simulink model "test_rfdcmask_zcu216"  (R2020b)
settings: Solver=VariableStepAuto  StartTime=0.0  StopTime=10.0  RelTol=1e-3
undefined symbols (not defined in the file): es1
libraries: xbsIndex_r4 x201, casper_library_misc x2
(part 1 of 4)
settings Model: Creator=mcb  LastModifiedBy=mcb
settings DataIOCC: ReturnWorkspaceOutputs=off
settings DebuggingCC: ArithmeticOperatorsInVariantConditions=warning
settings SFSimCC: CustomCodeUndefinedFunction=UseInterfaceOnly

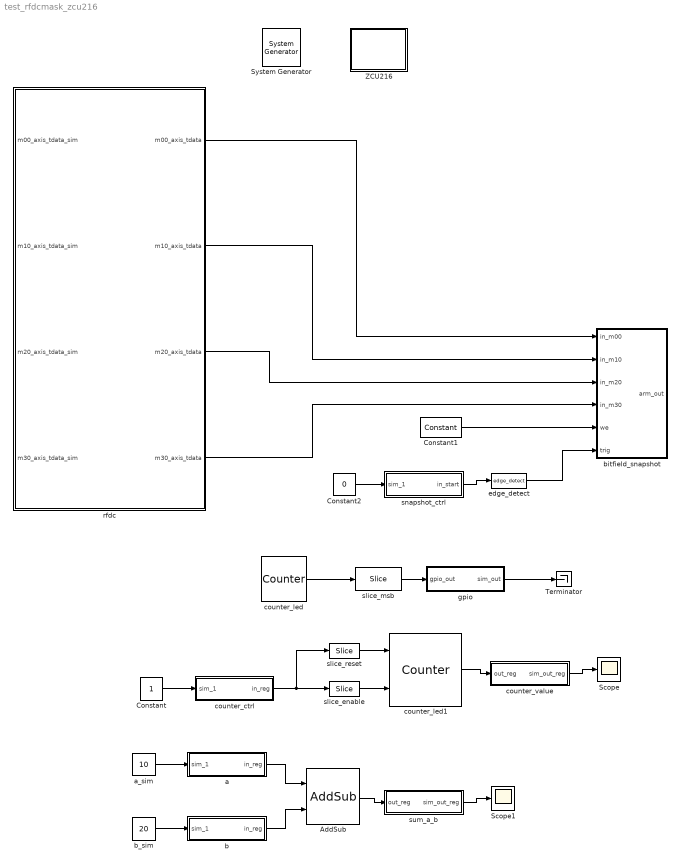
== system test_rfdcmask_zcu216 ==
  " System Generator" : xbsIndex_r4/ System Generator  Tag=genX  xilinxfamily=zynquplusRFSOCes1  part=xczu49dr  speed=-2-e-es1  package=ffvf1760  synthesis_tool=XST  clock_wrapper=Clock Enables  directory=/home/mcb/git/casper/mlib_devel/jasper_library/test_models/test_rfdcmask_zcu216/sysgen  proj_type=Vivado  Synth_file=Vivado Synthesis Defaults  Impl_file=Vivado Implementation Defaults  testbench=off  simulink_period=1  sysclk_period=4  dcm_input_clock_period=10  incr_netlist=off  trim_vbits=Everywhere in SubSystem  dbl_ovrd=According to Block Masks  core_generation=According to Block Masks  run_coregen=off  deprecated_control=off  eval_field=0  block_type=sysgen
  AddSub : xbsIndex_r4/AddSub  mode=Addition  use_carryin=off  use_carryout=off  en=off  latency=0  precision=User Defined  arith_type=Unsigned  n_bits=32  bin_pt=0  quantization=Truncate  overflow=Saturate  use_behavioral_HDL=off  hw_selection=Fabric  pipelined=off  dbl_ovrd=off  block_type=addsub
  Constant : Constant
  Constant1 : xbsIndex_r4/Constant  const=1.0  gui_display_data_type=Boolean  arith_type=Boolean  n_bits=16  bin_pt=14  preci_type=Single  exp_width=8  frac_width=24  explicit_period=on  period=1  equ=P=C  opselect=C  inp2=PCIN>>17  opr=+  inp1=P  carry=CIN  dbl_ovrd=off  block_type=constant
  Constant2 : Constant  Value=0
  Scope : Scope
  Scope1 : Scope
  Terminator : Terminator
  ZCU216 : Subsystem  Tag=xps:xsg  mask(xsg core config){hw_sys=ZCU216:xczu49dr, clk_src=adc_clk, clk_rate=250, pl_clk_rate=125, sample_period=1, synthesis_tool=XST}
      mask prompts: hw_sys "Hardware Platform"; clk_src "User IP Clock source"; clk_rate "User IP Clock Rate (MHz)"; pl_clk_rate "RFPLL PL Clock Rate (MHz)"; sample_period "Sample Period"; synthesis_tool "Synthesis Tool:"
      mask help:
      | The XSG Core Config block is used to configure the System Generator design
      | for the casper_xps toolflow. Settings here are used to configure the
      | Xilinx System Generator block parameters automatically, and control toolflow
      | script  execution. It needs to be at the top level of all designs being compiled
      | with the casper_xps toolflow.
      mask init:
      | xps_xsg_zcu216_conf_mask;
      mask Help: eval('xlWeb([getenv(''MLIB_ROOT''), ''\doc\html\sys_xsg_core_config\sys_xsg_core_config.html''])')
      mask TypeOptions hw_sys: ZCU216:xczu49dr
      mask TypeOptions clk_src: adc_clk
      mask TypeOptions synthesis_tool: Leonardo Spectrum | Synplify | Synplify Pro | XST
      mask Display: fprintf(['ZCU216']);
  a : Subsystem  Tag=xps:sw_reg  AncestorBlock=xps_library/Memory/software_register  mask(swreg){io_dir=From Processor, io_delay=0, init_val=0, sample_period=1, names=reg, bitwidths=32, bin_pts=0, arith_types=0, sim_port=on, show_format=off}
      mask prompts: io_dir "I/O direction"; io_delay "I/O delay"; init_val "Initial Value"; sample_period "Sample period"; names "Bitfield names [msb...lsb]"; bitwidths "Bitfield widths"; bin_pts "Bitfield binary pts"; arith_types "Bitfield types, ufix=0, fix=1, bool=2"; sim_port "Provide sim input/output?"; show_format "Print format string?"
      mask help: A 32-bit software-accessible register. Can be divided into bitfields of varying widths and types using the fields in the block mask.
      mask init:
      | swreg_init(gcb)
      settings: AttributesFormatString=1input
      mask TypeOptions io_dir: To Processor | From Processor
      mask Callback io_dir:
      | mask_enables = get_param(gcb, 'MaskEnables');
      | mask_names = get_param(gcb, 'MaskNames');
      | if strcmp(get_param(gcb, 'io_dir'), 'To Processor'),
      |     mask_enables{ismember(mask_names, 'sample_period')} = 'off';
      | else
      |     mask_enables{ismember(mask_names, 'sample_period')} = 'on';
      | end
      | set_param(gcb, 'MaskEnables', mask_enables);
      mask DialogControl ParameterTabVar0 Prompt: Setup
  a_sim : Constant  Value=10
  b : Subsystem  Tag=xps:sw_reg  AncestorBlock=xps_library/Memory/software_register  mask(swreg){io_dir=From Processor, io_delay=0, init_val=0, sample_period=1, names=reg, bitwidths=32, bin_pts=0, arith_types=0, sim_port=on, show_format=off}
      mask prompts: io_dir "I/O direction"; io_delay "I/O delay"; init_val "Initial Value"; sample_period "Sample period"; names "Bitfield names [msb...lsb]"; bitwidths "Bitfield widths"; bin_pts "Bitfield binary pts"; arith_types "Bitfield types, ufix=0, fix=1, bool=2"; sim_port "Provide sim input/output?"; show_format "Print format string?"
      mask help: A 32-bit software-accessible register. Can be divided into bitfields of varying widths and types using the fields in the block mask.
      mask init:
      | swreg_init(gcb)
      settings: AttributesFormatString=1input
      mask TypeOptions io_dir: To Processor | From Processor
      mask Callback io_dir:
      | mask_enables = get_param(gcb, 'MaskEnables');
      | mask_names = get_param(gcb, 'MaskNames');
      | if strcmp(get_param(gcb, 'io_dir'), 'To Processor'),
      |     mask_enables{ismember(mask_names, 'sample_period')} = 'off';
      | else
      |     mask_enables{ismember(mask_names, 'sample_period')} = 'on';
      | end
      | set_param(gcb, 'MaskEnables', mask_enables);
      mask DialogControl ParameterTabVar0 Prompt: Setup
  b_sim : Constant  Value=20
  bitfield_snapshot : Subsystem  Tag=casper:bitsnap  AncestorBlock=casper_library_scopes/bitfield_snapshot  mask(bitsnap){io_names=[m00 m10 m20 m30], io_widths=[16 16 16 16], io_bps=[0 0 0 0], io_types=[1 1 1 1], show_format=on, snap_storage=bram, snap_dram_dimm=2, snap_dram_clock=250, snap_nsamples=12, snap_data_width=64, snap_offset=off, snap_circap=off, snap_value=off, snap_ext_arm=off, snap_ext_circ=off, snap_provide_outputs=on, snap_use_dsp48=on, snap_delay=2, extra_names=[c d], extra_widths=[30 2], extra_bps=[0 0], extra_types=[0 0]}
      mask prompts: io_names "Names [msb...lsb]"; io_widths "Bitwidths [msb...lsb]"; io_bps "Binary pts [msb...lsb]"; io_types "Data types [msb...lsb], ufix=0, fix=1, bool=2"; show_format "Print format string?"; snap_storage "Storage medium"; snap_dram_dimm "DRAM dimm"; snap_dram_clock "DRAM clock rate"; snap_nsamples "Number of Samples (2^?)"; snap_data_width "Data width"; snap_offset "Start delay support"; snap_circap "Circular capture support"; snap_value "Extra value capture support"; snap_ext_arm "External arm support"; snap_ext_circ "External circular capture support"; snap_provide_outputs "Provide outputs"; snap_use_dsp48 "Use DSP48s to implement counters"; snap_delay "Pre-snapshot delay"; extra_names "Names [msb...lsb]"; extra_widths "Widths [msb...lsb]"; extra_bps "Binary pts [msb...lsb]"; extra_types "Data types [msb...lsb], ufix=0, fix=1, bool=2"
      mask help:
      | A wrapped snapshot block. Allows specification of inputs to a snapblock word so the toolflow can automatically set up the scope.
      | See documentation for snapshot for explanation of parameters.
      mask init:
      | bitsnap_init(gcb);
      settings: AttributesFormatString=|
      | snap(4):f16.0,f16.0,f16.0,f16.0 = 64 bits\n64 wide, 4096 deep
      | debugID: 125644504
      mask TypeOptions snap_storage: bram | dram
      mask Callback snap_storage: bitsnap_callback();
      mask TypeOptions snap_dram_dimm: 1 | 2 | 3 | 4
      mask TypeOptions snap_dram_clock: 200 | 250 | 266 | 300 | 333
      mask TypeOptions snap_data_width: 8 | 16 | 32 | 64 | 128
      mask Callback snap_value: bitsnap_callback();
      mask Callback snap_ext_arm: bitsnap_callback();
      mask Callback snap_ext_circ: bitsnap_callback();
      mask Callback snap_provide_outputs: bitsnap_callback();
      mask DialogControl ParameterTabVar0 Prompt: Inputs
      mask DialogControl ParameterTabVar01 Prompt: Snapshot
      mask DialogControl ParameterTabVar012 Prompt: Extra Value
  counter_ctrl : Subsystem  Tag=xps:sw_reg  AncestorBlock=xps_library/Memory/software_register  mask(swreg){io_dir=From Processor, io_delay=0, init_val=0, sample_period=1, names=reg, bitwidths=32, bin_pts=0, arith_types=0, sim_port=on, show_format=off}
      mask prompts: io_dir "I/O direction"; io_delay "I/O delay"; init_val "Initial Value"; sample_period "Sample period"; names "Bitfield names [msb...lsb]"; bitwidths "Bitfield widths"; bin_pts "Bitfield binary pts"; arith_types "Bitfield types, ufix=0, fix=1, bool=2"; sim_port "Provide sim input/output?"; show_format "Print format string?"
      mask help: A 32-bit software-accessible register. Can be divided into bitfields of varying widths and types using the fields in the block mask.
      mask init:
      | swreg_init(gcb)
      settings: AttributesFormatString=1input
      mask TypeOptions io_dir: To Processor | From Processor
      mask Callback io_dir:
      | mask_enables = get_param(gcb, 'MaskEnables');
      | mask_names = get_param(gcb, 'MaskNames');
      | if strcmp(get_param(gcb, 'io_dir'), 'To Processor'),
      |     mask_enables{ismember(mask_names, 'sample_period')} = 'off';
      | else
      |     mask_enables{ismember(mask_names, 'sample_period')} = 'on';
      | end
      | set_param(gcb, 'MaskEnables', mask_enables);
      mask DialogControl ParameterTabVar0 Prompt: Setup
  counter_led : xbsIndex_r4/Counter  cnt_type=Free Running  cnt_to=Inf  operation=Up  start_count=0  cnt_by_val=1  arith_type=Unsigned  n_bits=28  bin_pt=0  load_pin=off  rst=off  en=off  explicit_period=on  period=1  use_behavioral_HDL=off  implementation=Fabric  dbl_ovrd=off  block_type=counter
  counter_led1 : xbsIndex_r4/Counter  cnt_type=Free Running  cnt_to=Inf  operation=Up  start_count=0  cnt_by_val=1  arith_type=Unsigned  n_bits=32  bin_pt=0  load_pin=off  rst=on  en=on  explicit_period=on  period=1  use_behavioral_HDL=off  implementation=Fabric  dbl_ovrd=off  block_type=counter
  counter_value : Subsystem  Tag=xps:sw_reg  AncestorBlock=xps_library/Memory/software_register  mask(swreg){io_dir=To Processor, io_delay=0, init_val=0, sample_period=1, names=reg, bitwidths=32, bin_pts=0, arith_types=0, sim_port=on, show_format=off}
      mask prompts: io_dir "I/O direction"; io_delay "I/O delay"; init_val "Initial Value"; sample_period "Sample period"; names "Bitfield names [msb...lsb]"; bitwidths "Bitfield widths"; bin_pts "Bitfield binary pts"; arith_types "Bitfield types, ufix=0, fix=1, bool=2"; sim_port "Provide sim input/output?"; show_format "Print format string?"
      mask help: A 32-bit software-accessible register. Can be divided into bitfields of varying widths and types using the fields in the block mask.
      mask init:
      | swreg_init(gcb)
      settings: AttributesFormatString=1output
      mask TypeOptions io_dir: To Processor | From Processor
      mask Callback io_dir:
      | mask_enables = get_param(gcb, 'MaskEnables');
      | mask_names = get_param(gcb, 'MaskNames');
      | if strcmp(get_param(gcb, 'io_dir'), 'To Processor'),
      |     mask_enables{ismember(mask_names, 'sample_period')} = 'off';
      | else
      |     mask_enables{ismember(mask_names, 'sample_period')} = 'on';
      | end
      | set_param(gcb, 'MaskEnables', mask_enables);
      mask DialogControl ParameterTabVar0 Prompt: Setup
  edge_detect : casper_library_misc/edge_detect  edge=Rising  polarity=Active High  x_in=[0 0.08 0.08 0.16 0.16 0.24 0.24 0.32 0.32 0.4]  y_in="[-1 -1  1  1  1  1  1  1  1  1]"  x_out=[0.6 0.68 0.68 0.76 0.76 0.84 0.84 0.92 0.92 1]  y_out="[-1 -1  1  1 -1 -1 -1 -1 -1 -1]"
  gpio : Subsystem  Tag=xps:gpio  AncestorBlock=xps_library/IO/gpio  mask(gpio){io_group_params_forwarded=on, io_group=ROACH2:led, io_group_real=led, io_group_custom=0, io_dir=out, arith_type=Boolean, bitwidth=1, bin_pt=0, bit_index=0, sample_period=1, use_single_ended=off, use_ddr=off, reg_iob=on, reg_clk_phase=0, termination=None}
      mask prompts: io_group_params_forwarded "Have the io_group params been forwarded yet?"; io_group "I/O group"; io_group_real "I/O group"; io_group_custom "Custom I/O group"; io_dir "I/O direction"; arith_type "Data Type"; bitwidth "Data bitwidth"; bin_pt "Data binary point"; bit_index "GPIO bit index"; sample_period "Sample period"; use_single_ended "Use as single-ended"; use_ddr "Use DDR"; reg_iob "Pack register in the pad"; reg_clk_phase "Register clock phase"; termination "Termination method"
      mask help:
      | GPIO interfaces for CASPER hardware.
      |
      | For usage of LEDs on SKARAB boards, please note that the board will boot into 'BSP mode' by default. To change the control of the Front Panel LEDs to your design, execute the command 'control_front_panel_leds_write()' on your SKARAB CASPERFPGA object via the transport layer.
      |
      | For more information please click help below.
      mask init:
      | gpio_mask;
      mask Help: If you've come here for more help, unfortunately I'm going to direct you to the ska-sa/casperfpga wiki. The documentation at https://github.com/ska-sa/casperfpga/wiki/SKARAB-Front-Panel-LED-Manager outlines the signals that are used to control the SKARAB's Front Panel LEDs by default, and the mechanism by which you can switch control to the DSP Design.
      mask TypeOptions io_group: ROACH:aux0_clk | ROACH:aux1_clk | ROACH:led | ROACH:gpioa | ROACH:gpioa_oe_n | ROACH:gpiob | ROACH:gpiob_oe_n | ROACH:qsh | ROACH:zdok0 | ROACH:zdok1 | ROACH2:aux_clk | ROACH2:led | ROACH2:gpio | ROACH2:qsh | ROACH2:sync_in | ROACH2:sync_out | ROACH2:zdok0 | ROACH2:zdok1 | custom:custom
      mask TypeOptions io_group_real: led | gpio | sync_in | sync_out | zdok0 | zdok1 | aux_clk_diff | custom
      mask Callback io_group_real:
      | if ~isempty(find(strcmp(get_param(gcb, 'io_group_real'), {'zdok0' 'zdok1' 'sync_in' 'sync_out'})))
      |     set_param(gcb, 'MaskEnables', {'off', 'off', 'on','off','on','on','on','on','on','on','on','on','on','on','on'});
      | elseif ~isempty(find(strcmp(get_param(gcb, 'io_group_real'), {'custom'})))
      |     set_param(gcb, 'MaskEnables', {'off', 'off', 'on','on','on','on','on','on','on','on','off','on','on','on','on'});
      | else
      |     set_param(gcb, 'MaskEnables', {'off', 'off', 'on','off','on','on','on','on','on','on','off','on','on','on','on'});
      | end
      mask TypeOptions io_dir: in | out
      mask Callback io_dir:
      | if ~isempty(find(strcmp(get_param(gcb, 'io_group_real'), {'zdok0' 'zdok1' 'sync_in' 'sync_out'})))
      |     set_param(gcb, 'MaskVisibilities', {'off', 'off','on','on','on','on','on','on','on','on','on','on','on','on','on'});
      | else
      |     set_param(gcb, 'MaskVisibilities', {'off', 'off','on','on','on','on','on','on','on','on','off','on','on','on','on'});
      | end
      mask TypeOptions arith_type: Boolean | Unsigned | Signed  (2's comp)
      mask Callback use_ddr:
      | if strcmp(get_param(gcb,'use_ddr'),'on')
      |     set_param(gcb,'reg_iob','on');
      |     set_param(gcb,'MaskEnables', {'off' 'off' 'on' 'on' 'on' 'on' 'on' 'on' 'on' 'on' 'on' 'on' 'off' 'on' 'on'});
      | else
      |     set_param(gcb,'MaskEnables', {'off' 'off' 'on' 'on' 'on' 'on' 'on' 'on' 'on' 'on' 'on' 'on' 'on' 'on' 'on'});
      | end
      mask TypeOptions reg_clk_phase: 0 | 90 | 180 | 270
      mask TypeOptions termination: None | Pullup | Pulldown
  rfdc : Subsystem  Tag=xps:rfdc  mask(Xilinx RF Data Converter){Tile224_enable=on, Tile225_enable=on, Tile226_enable=on, Tile227_enable=on, enable_mts=off, sample_rate=2000, clk_out=250, enable_pll=on, ref_clk=250, axi_stream_clk=250, QT_adc0_enable=on, QT_adc0_digital_output=Real, QT_adc0_dec_mode=8x, QT_adc0_sample_per_cycle=1, QT_adc0_req_axis_clk=250, QT_adc0_mixer_type=Bypassed, QT_adc0_mixer_mode=Real -> Real, QT_adc1_enable=off, QT_adc1_digital_output=Real, QT_adc1_dec_mode=8x, QT_adc1_sample_per_cycle=1, QT_adc1_req_axis_clk=250, QT_adc1_mixer_type=Fine, QT_adc1_mixer_mode=Real -> I/Q, QT_adc2_enable=off, QT_adc2_digital_output=Real, QT_adc2_dec_mode=8x, QT_adc2_sample_per_cycle=1, QT_adc2_req_axis_clk=250, QT_adc2_mixer_type=Bypassed, QT_adc2_mixer_mode=Real -> Real, QT_adc3_enable=off, QT_adc3_digital_output=Real, QT_adc3_dec_mode=8x, QT_adc3_sample_per_cycle=1, QT_adc3_req_axis_clk=250, QT_adc3_mixer_type=Fine, QT_adc3_mixer_mode=Real -> I/Q, DT_adc0_enable=on, DT_adc0_digital_output=Real, DT_adc0_dec_mode=2x, DT_adc0_sample_per_cycle=8, DT_adc0_req_axis_clk=0, DT_adc0_mixer_type=Bypassed, DT_adc0_mixer_mode=Real -> Real, DT_adc1_enable=on, DT_adc1_digital_output=Real, DT_adc1_dec_mode=2x, DT_adc1_sample_per_cycle=8, DT_adc1_req_axis_clk=0, DT_adc1_mixer_type=Bypassed, DT_adc1_mixer_mode=Real -> Real}
      mask prompts: Tile224_enable "Tile 224"; Tile225_enable "Tile 225"; Tile226_enable "Tile 226"; Tile227_enable "Tile 227"; enable_mts "Enable Multi-Tile Sync"; sample_rate "Sampling Rate (Msps)"; clk_out "Clock Out (MHz)"; enable_pll "Enable Tile PLLs"; ref_clk "Reference Clock (MHz)"; axi_stream_clk "Required AXI4-Stream Clock (MHz)"; QT_adc0_enable "Enable ADC"; QT_adc0_digital_output "Digital Output Data"; QT_adc0_dec_mode "Decimation Mode"; QT_adc0_sample_per_cycle "Samples per AXI4-Stream Cycle"; QT_adc0_mixer_type "Mixer Type"; QT_adc0_mixer_mode "Mixer Mode"; QT_adc1_enable "Enable ADC"; QT_adc1_digital_output "Digital Output Data"; QT_adc1_dec_mode "Decimation Mode"; QT_adc1_sample_per_cycle "Samples per AXI4-Stream Cycle"; QT_adc1_mixer_type "Mixer Type"; QT_adc1_mixer_mode "Mixer Mode"; QT_adc2_enable "Enable ADC"; QT_adc2_digital_output "Digital Output Data"; QT_adc2_dec_mode "Decimation Mode"; QT_adc2_sample_per_cycle "Samples per AXI4-Stream Cycle"; QT_adc2_mixer_type "Mixer Type"; QT_adc2_mixer_mode "Mixer Mode"; QT_adc3_enable "Enable ADC"; QT_adc3_digital_output "Digital Output Data"; QT_adc3_dec_mode "Decimation Mode"; QT_adc3_sample_per_cycle "Samples per AXI4-Stream Cycle"; QT_adc3_mixer_type "Mixer Type"; QT_adc3_mixer_mode "Mixer Mode"; DT_adc0_enable "Enable ADC"; DT_adc0_digital_output "Digital Output Data"; DT_adc0_dec_mode "Decimation Mode"; DT_adc0_sample_per_cycle "Samples per AXI4-Stream Cycle"; DT_adc0_mixer_type "Mixer Type"; DT_adc0_mixer_mode "Mixer Mode"; DT_adc1_enable "Enable ADC"; DT_adc1_digital_output "Digital Output Data"; DT_adc1_dec_mode "Decimation Mode"; DT_adc1_sample_per_cycle "Samples per AXI4-Stream Cycle"; DT_adc1_mixer_type "Mixer Type"; DT_adc1_mixer_mode "Mixer Mode"
      mask help: I am my mask description!
      mask init:
      | rfdc_mask(gcb);
      mask Help: eval('xlWeb([getenv(''MLIB_ROOT''), ''\doc\html\adc_zcu111\adc_zcu111.html''])')
      mask Callback Tile224_enable: enable_mts_opt(gcb);
      mask Callback sample_rate: update_rfdc_clocking(gcb);
      mask TypeOptions clk_out: 250 | 125 | 62.5 | 31.25
      mask Callback enable_pll:
      | %update_rfdc_clocking(gcb);
      | update_pll(gcb);
      mask TypeOptions ref_clk: 923.077 | 857.143 | 800 | 750 | 705.882 | 666.667 | 631.579 | 600 | 571.429 | 545.455 | 521.739 | 500 | 480 | 461.538 | 444.444 | 428.571 | 413.793 | 400 | 387.097 | 375 | 363.636 | 352.941 | 342.857 | 333.333 | 324.324 | 315.789 | 307.692 | 300 | 292.683 | 285.714 | 279.07 | 272.727 | 266.667 | 260.87 | 255.319 | 250 | 244.898 | 240 | 235.294 | 230.769 | 226.415 | 222.222 | 218.182 | 214.286 | 210.526 | 206.897 | 203.39 | 200 | 196.721 | 193.548 | 190.476 | 187.5 | 184.615 | 181.818 | 179.104 | 176.471 | 173.913 | 171.429 | 169.014 | 166.667 | 164.384 | 162.162 | 160 | 157.895 | 155.844 | 153.846 | 151.899 | 150 | 148.148 | 146.341 | 144.578 | 142.857 | 141.176 | 139.535 | 137.931 | 136.364 | 134.831 | 133.333 | 131.868 | 130.435 | 129.032 | 127.66 | 126.316 | 125 | 123.711 | 122.449 | 121.212 | 120 | 118.812 | 117.647 | 116.505 | 115.385 | 114.286 | 113.208 | 112.15 | 111.111 | 110.092 | 109.091 | 108.108 | 107.143 | 106.195 | 105.263 | 104.348 | 103.448 | 102.564
      mask Callback QT_adc0_enable: enable_adc_opt(gcb);
      mask TypeOptions QT_adc0_digital_output: Real | I/Q
      mask Callback QT_adc0_digital_output:
      | validate_digital_data(gcb);
      | update_axis_clk(gcb);
      mask TypeOptions QT_adc0_dec_mode: 1x | 2x | 4x | 8x
      mask Callback QT_adc0_dec_mode: update_axis_clk(gcb);
      mask TypeOptions QT_adc0_sample_per_cycle: 1 | 2 | 3 | 4 | 5 | 6 | 7 | 8 | 9 | 10 | 11 | 12
      mask Callback QT_adc0_sample_per_cycle:
      | %update_axis_clk(gcb);
      | update_axis_clk_label(gcb);
      mask TypeOptions QT_adc0_mixer_type: Bypassed
      mask TypeOptions QT_adc0_mixer_mode: Real -> Real
      mask Callback QT_adc0_mixer_mode: mixer_callback(gcb);
      mask Callback QT_adc1_enable: enable_adc_opt(gcb);
      mask TypeOptions QT_adc1_digital_output: Real | I/Q
      mask Callback QT_adc1_digital_output:
      | validate_digital_data(gcb);
      | update_axis_clk(gcb);
      mask TypeOptions QT_adc1_dec_mode: 1x | 2x | 4x | 8x
      mask Callback QT_adc1_dec_mode: update_axis_clk(gcb);
      mask TypeOptions QT_adc1_sample_per_cycle: 1 | 2 | 3 | 4 | 5 | 6 | 7 | 8 | 9 | 10 | 11 | 12
      mask Callback QT_adc1_sample_per_cycle: update_axis_clk_label(gcb);
      mask TypeOptions QT_adc1_mixer_type: Fine | Coarse
      mask TypeOptions QT_adc1_mixer_mode: Real -> I/Q
      mask Callback QT_adc2_enable: enable_adc_opt(gcb);
      mask TypeOptions QT_adc2_digital_output: Real | I/Q
      mask Callback QT_adc2_digital_output:
      | validate_digital_data(gcb);
      | update_axis_clk(gcb);
      mask TypeOptions QT_adc2_dec_mode: 1x | 2x | 4x | 8x
      mask Callback QT_adc2_dec_mode: update_axis_clk(gcb);
      mask TypeOptions QT_adc2_sample_per_cycle: 1 | 2 | 3 | 4 | 5 | 6 | 7 | 8 | 9 | 10 | 11 | 12
      mask Callback QT_adc2_sample_per_cycle: update_axis_clk_label(gcb);
      mask TypeOptions QT_adc2_mixer_type: Bypassed
      mask TypeOptions QT_adc2_mixer_mode: Real -> Real
      mask Callback QT_adc3_enable: enable_adc_opt(gcb);
      mask TypeOptions QT_adc3_digital_output: Real | I/Q
      mask Callback QT_adc3_digital_output:
      | validate_digital_data(gcb);
      | update_axis_clk(gcb);
      mask TypeOptions QT_adc3_dec_mode: 1x | 2x | 4x | 8x
      mask Callback QT_adc3_dec_mode: update_axis_clk(gcb);
      mask TypeOptions QT_adc3_sample_per_cycle: 1 | 2 | 3 | 4 | 5 | 6 | 7 | 8 | 9 | 10 | 11 | 12
      mask Callback QT_adc3_sample_per_cycle: update_axis_clk_label(gcb);
      mask TypeOptions QT_adc3_mixer_type: Fine | Coarse
      mask TypeOptions QT_adc3_mixer_mode: Real -> I/Q
      mask Callback DT_adc0_enable: enable_adc_opt(gcb);
      mask TypeOptions DT_adc0_digital_output: Real | I/Q
      mask Callback DT_adc0_digital_output:
      | validate_digital_data(gcb);
      | update_axis_clk(gcb);
      mask TypeOptions DT_adc0_dec_mode: 1x | 2x | 4x | 8x
      mask Callback DT_adc0_dec_mode: update_axis_clk(gcb);
      mask TypeOptions DT_adc0_sample_per_cycle: 1 | 2 | 3 | 4 | 5 | 6 | 7 | 8
      mask Callback DT_adc0_sample_per_cycle:
      | %update_axis_clk(gcb);
      | update_axis_clk_label(gcb);
      mask TypeOptions DT_adc0_mixer_type: Bypassed | Coarse | Fine
      mask TypeOptions DT_adc0_mixer_mode: Real -> Real | Real -> I/Q | I/Q -> I/Q
      mask Callback DT_adc0_mixer_mode: mixer_callback(gcb);
      mask Callback DT_adc1_enable: enable_adc_opt(gcb);
      mask TypeOptions DT_adc1_digital_output: Real | I/Q
      mask Callback DT_adc1_digital_output:
      | validate_digital_data(gcb);
      | update_axis_clk(gcb);
      mask TypeOptions DT_adc1_dec_mode: 1x | 2x | 4x | 8x
      mask Callback DT_adc1_dec_mode: update_axis_clk(gcb);
      mask TypeOptions DT_adc1_sample_per_cycle: 1 | 2 | 3 | 4 | 5 | 6 | 7 | 8
      mask Callback DT_adc1_sample_per_cycle:
      | %update_axis_clk(gcb);
      | update_axis_clk_label(gcb);
      mask TypeOptions DT_adc1_mixer_type: Bypassed | Coarse | Fine
      mask TypeOptions DT_adc1_mixer_mode: Real -> Real | Real -> I/Q | I/Q -> I/Q
      mask Callback DT_adc1_mixer_mode: mixer_callback(gcb);
      mask DialogControl TileSelect Prompt: ADC Tiles
      mask DialogControl pll_clocking_config_224 Prompt: Clocking and PLL Configuration
      mask DialogControl QuadTileConfig Prompt: Quad Tile Configuration
      mask DialogControl ADCPair01 Prompt: ADC Pair 0,1
      mask DialogControl QT_adc0 Prompt: ADC 0
      mask DialogControl QT_adc0_DataSettings Prompt: Data Settings
      mask DialogControl QT_adc0_req_axis_clk_label Prompt: Required AXI4-Stream clock:
      mask DialogControl QT_adc0_MixerSettings Prompt: MIxer Settings
      mask DialogControl QT_adc1 Prompt: ADC 1
      mask DialogControl QT_adc1_DataSettings Prompt: Data Settings
      mask DialogControl QT_adc1_req_axis_clk_label Prompt: Required AXI4-Stream clock:
      mask DialogControl QT_adc1_MixerSettings Prompt: MIxer Settings
      mask DialogControl ADCPair23 Prompt: ADC Pair 2,3
      mask DialogControl QT_adc2 Prompt: ADC 2
      mask DialogControl QT_adc2_DataSettings Prompt: Data Settings
      mask DialogControl QT_adc2_req_axis_clk_label Prompt: Required AXI4-Stream clock:
      mask DialogControl QT_adc2_MixerSettings Prompt: MIxer Settings
      mask DialogControl QT_adc3 Prompt: ADC 3
      mask DialogControl QT_adc3_DataSettings Prompt: Data Settings
      mask DialogControl QT_adc3_req_axis_clk_label Prompt: Required AXI4-Stream clock:
      mask DialogControl QT_adc3_MixerSettings Prompt: MIxer Settings
      mask DialogControl DualTileConfig Prompt: Dual Tile Configuration
      mask DialogControl DT_adc0 Prompt: ADC 0
      mask DialogControl DT_adc0_DataSettings Prompt: Data Settings
      mask DialogControl DT_adc0_req_axis_clk_label Prompt: Required AXI4-Stream clock:
      mask DialogControl DT_adc0_MixerSettings Prompt: MIxer Settings
      mask DialogControl DT_adc1 Prompt: ADC 1
      mask DialogControl DT_adc1_DataSettings Prompt: Data Settings
      mask DialogControl DT_adc1_req_axis_clk_label Prompt: Required AXI4-Stream clock:
      mask DialogControl DT_adc1_MixerSettings Prompt: MIxer Settings
  slice_enable : xbsIndex_r4/Slice  nbits=1  boolean_output=on  mode=Lower Bit Location + Width  bit1=0  base1=MSB of Input  bit0=0  base0=LSB of Input  dbl_ovrd=off  block_type=slice
  slice_msb : xbsIndex_r4/Slice  nbits=1  boolean_output=off  mode=Upper Bit Location + Width  bit1=0  base1=MSB of Input  bit0=0  base0=LSB of Input  dbl_ovrd=off  block_type=slice
  slice_reset : xbsIndex_r4/Slice  nbits=1  boolean_output=on  mode=Lower Bit Location + Width  bit1=0  base1=MSB of Input  bit0=1  base0=LSB of Input  dbl_ovrd=off  block_type=slice
  snapshot_ctrl : Subsystem  Tag=xps:sw_reg  AncestorBlock=xps_library/Memory/software_register  mask(swreg){io_dir=From Processor, io_delay=0, init_val=0, sample_period=1, names=[start], bitwidths=1, bin_pts=0, arith_types=2, sim_port=on, show_format=on}
      mask prompts: io_dir "I/O direction"; io_delay "I/O delay"; init_val "Initial Value"; sample_period "Sample period"; names "Bitfield names [msb...lsb]"; bitwidths "Bitfield widths"; bin_pts "Bitfield binary pts"; arith_types "Bitfield types, ufix=0, fix=1, bool=2"; sim_port "Provide sim input/output?"; show_format "Print format string?"
      mask help: A 32-bit software-accessible register. Can be divided into bitfields of varying widths and types using the fields in the block mask.
      mask init:
      | swreg_init(gcb)
      settings: AttributesFormatString=1input:b = 1 bits
      mask TypeOptions io_dir: To Processor | From Processor
      mask Callback io_dir:
      | mask_enables = get_param(gcb, 'MaskEnables');
      | mask_names = get_param(gcb, 'MaskNames');
      | if strcmp(get_param(gcb, 'io_dir'), 'To Processor'),
      |     mask_enables{ismember(mask_names, 'sample_period')} = 'off';
      | else
      |     mask_enables{ismember(mask_names, 'sample_period')} = 'on';
      | end
      | set_param(gcb, 'MaskEnables', mask_enables);
      mask DialogControl ParameterTabVar0 Prompt: Setup
  sum_a_b : Subsystem  Tag=xps:sw_reg  AncestorBlock=xps_library/Memory/software_register  mask(swreg){io_dir=To Processor, io_delay=0, init_val=0, sample_period=1, names=reg, bitwidths=32, bin_pts=0, arith_types=0, sim_port=on, show_format=off}
      mask prompts: io_dir "I/O direction"; io_delay "I/O delay"; init_val "Initial Value"; sample_period "Sample period"; names "Bitfield names [msb...lsb]"; bitwidths "Bitfield widths"; bin_pts "Bitfield binary pts"; arith_types "Bitfield types, ufix=0, fix=1, bool=2"; sim_port "Provide sim input/output?"; show_format "Print format string?"
      mask help: A 32-bit software-accessible register. Can be divided into bitfields of varying widths and types using the fields in the block mask.
      mask init:
      | swreg_init(gcb)
      settings: AttributesFormatString=1output
      mask TypeOptions io_dir: To Processor | From Processor
      mask Callback io_dir:
      | mask_enables = get_param(gcb, 'MaskEnables');
      | mask_names = get_param(gcb, 'MaskNames');
      | if strcmp(get_param(gcb, 'io_dir'), 'To Processor'),
      |     mask_enables{ismember(mask_names, 'sample_period')} = 'off';
      | else
      |     mask_enables{ismember(mask_names, 'sample_period')} = 'on';
      | end
      | set_param(gcb, 'MaskEnables', mask_enables);
      mask DialogControl ParameterTabVar0 Prompt: Setup
  wires:
  slice_reset/1 -> counter_led1/1
  Constant/1 -> counter_ctrl/1(sim_1)
  counter_ctrl/1(in_reg) -> slice_reset/1, slice_enable/1
  counter_led1/1 -> counter_value/1(out_reg)
  slice_enable/1 -> counter_led1/2
  gpio/1(sim_out) -> Terminator/1
  slice_msb/1 -> gpio/1(gpio_out)
  counter_led/1 -> slice_msb/1
  counter_value/1(sim_out_reg) -> Scope/1
  a_sim/1 -> a/1(sim_1)
  AddSub/1 -> sum_a_b/1(out_reg)
  b_sim/1 -> b/1(sim_1)
  b/1(in_reg) -> AddSub/2
  a/1(in_reg) -> AddSub/1
  sum_a_b/1(sim_out_reg) -> Scope1/1
  edge_detect/1 -> bitfield_snapshot/6(trig)
  Constant1/1 -> bitfield_snapshot/5(we)
  snapshot_ctrl/1(in_start) -> edge_detect/1
  Constant2/1 -> snapshot_ctrl/1(sim_1)
  rfdc/1(m00_axis_tdata) -> bitfield_snapshot/1(in_m00)
  rfdc/2(m10_axis_tdata) -> bitfield_snapshot/2(in_m10)
  rfdc/3(m20_axis_tdata) -> bitfield_snapshot/3(in_m20)
  rfdc/4(m30_axis_tdata) -> bitfield_snapshot/4(in_m30)

== system test_rfdcmask_zcu216/ZCU216 ==

== system test_rfdcmask_zcu216/a ==
  sim_1 : Inport
  convert1_1 : DataTypeConversion  OutDataTypeStr=fixdt('ufix32_En0')  LockScale=on
  convert2_1 : DataTypeConversion  OutDataTypeStr=fixdt('ufix32_En0')  ConvertRealWorld=Stored Integer (SI)  LockScale=on
  gain_1 : Gain
  io_delay : xbsIndex_r4/Delay  rst=off  infoeditControl=Selection of Reset will increase slice count due to use of real FFs and instead of SRLs  en=off  latency=0  reg_retiming=on  dbl_ovrd=off  block_type=delay
  reint1 : xbsIndex_r4/Reinterpret  force_arith_type=on  arith_type=Unsigned  force_bin_pt=on  bin_pt=0  block_type=reinterpret
  slice_reg : xbsIndex_r4/Slice  nbits=32  boolean_output=off  mode=Lower Bit Location + Width  bit1=0  base1=MSB of Input  bit0=0  base0=LSB of Input  dbl_ovrd=off  block_type=slice
  test_rfdcmask_zcu216_a_user_data_out : xbsIndex_r4/Gateway In  gui_display_data_type=Fixed-point  arith_type=Unsigned  n_bits=32  bin_pt=0  preci_type=Single  exp_width=8  frac_width=24  rows=1  columns=1  quantization="Round  (unbiased: +/- Inf)"  overflow=Saturate  period=1  UseAsADC=off  ADCChannel='1'  interface=None  automatic_assignment=on  address_offset=hex2dec('00')  intf_name=''  intf_description=''  default_value=0  timing_constraint=None  locs_specified=off  LOCs={}  io_standard={}  inherit_from_input=off  hdl_port=on  dbl_ovrd=off  block_type=gatewayin
  in_reg : Outport  VectorParamsAs1DForOutWhenUnconnected=off
  wires:
  test_rfdcmask_zcu216_a_user_data_out/1 -> io_delay/1
  sim_1/1 -> convert1_1/1
  convert1_1/1 -> convert2_1/1
  convert2_1/1 -> gain_1/1
  gain_1/1 -> test_rfdcmask_zcu216_a_user_data_out/1
  io_delay/1 -> slice_reg/1
  slice_reg/1 -> reint1/1
  reint1/1 -> in_reg/1

== system test_rfdcmask_zcu216/b ==
  sim_1 : Inport
  convert1_1 : DataTypeConversion  OutDataTypeStr=fixdt('ufix32_En0')  LockScale=on
  convert2_1 : DataTypeConversion  OutDataTypeStr=fixdt('ufix32_En0')  ConvertRealWorld=Stored Integer (SI)  LockScale=on
  gain_1 : Gain
  io_delay : xbsIndex_r4/Delay  rst=off  infoeditControl=Selection of Reset will increase slice count due to use of real FFs and instead of SRLs  en=off  latency=0  reg_retiming=on  dbl_ovrd=off  block_type=delay
  reint1 : xbsIndex_r4/Reinterpret  force_arith_type=on  arith_type=Unsigned  force_bin_pt=on  bin_pt=0  block_type=reinterpret
  slice_reg : xbsIndex_r4/Slice  nbits=32  boolean_output=off  mode=Lower Bit Location + Width  bit1=0  base1=MSB of Input  bit0=0  base0=LSB of Input  dbl_ovrd=off  block_type=slice
  test_rfdcmask_zcu216_b_user_data_out : xbsIndex_r4/Gateway In  gui_display_data_type=Fixed-point  arith_type=Unsigned  n_bits=32  bin_pt=0  preci_type=Single  exp_width=8  frac_width=24  rows=1  columns=1  quantization="Round  (unbiased: +/- Inf)"  overflow=Saturate  period=1  UseAsADC=off  ADCChannel='1'  interface=None  automatic_assignment=on  address_offset=hex2dec('00')  intf_name=''  intf_description=''  default_value=0  timing_constraint=None  locs_specified=off  LOCs={}  io_standard={}  inherit_from_input=off  hdl_port=on  dbl_ovrd=off  block_type=gatewayin
  in_reg : Outport  VectorParamsAs1DForOutWhenUnconnected=off
  wires:
  test_rfdcmask_zcu216_b_user_data_out/1 -> io_delay/1
  sim_1/1 -> convert1_1/1
  convert1_1/1 -> convert2_1/1
  convert2_1/1 -> gain_1/1
  gain_1/1 -> test_rfdcmask_zcu216_b_user_data_out/1
  io_delay/1 -> slice_reg/1
  slice_reg/1 -> reint1/1
  reint1/1 -> in_reg/1

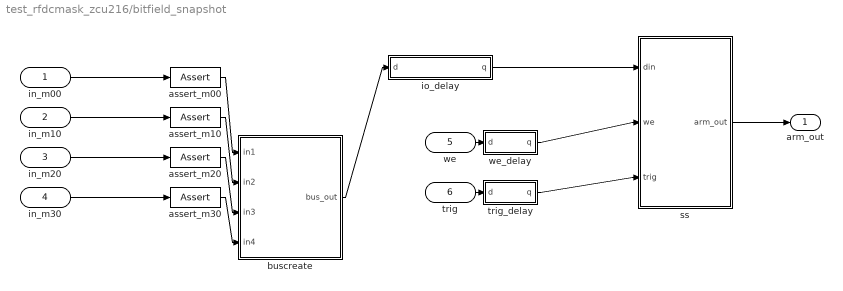
== system test_rfdcmask_zcu216/bitfield_snapshot ==
  in_m00 : Inport
  in_m10 : Inport  Port=2
  in_m20 : Inport  Port=3
  in_m30 : Inport  Port=4
  we : Inport  Port=5
  trig : Inport  Port=6
  assert_m00 : xbsIndex_r4/Assert  assert_type=on  type_source=Explicitly  gui_display_data_type=Fixed-point  arith_type="Signed  (2's comp)"  n_bits=16  bin_pt=0  preci_type=Single  exp_width=8  frac_width=24  assert_rate=off  rate_source=Explicitly  period=1  output_port=on  block_type=assert
  assert_m10 : xbsIndex_r4/Assert  assert_type=on  type_source=Explicitly  gui_display_data_type=Fixed-point  arith_type="Signed  (2's comp)"  n_bits=16  bin_pt=0  preci_type=Single  exp_width=8  frac_width=24  assert_rate=off  rate_source=Explicitly  period=1  output_port=on  block_type=assert
  assert_m20 : xbsIndex_r4/Assert  assert_type=on  type_source=Explicitly  gui_display_data_type=Fixed-point  arith_type="Signed  (2's comp)"  n_bits=16  bin_pt=0  preci_type=Single  exp_width=8  frac_width=24  assert_rate=off  rate_source=Explicitly  period=1  output_port=on  block_type=assert
  assert_m30 : xbsIndex_r4/Assert  assert_type=on  type_source=Explicitly  gui_display_data_type=Fixed-point  arith_type="Signed  (2's comp)"  n_bits=16  bin_pt=0  preci_type=Single  exp_width=8  frac_width=24  assert_rate=off  rate_source=Explicitly  period=1  output_port=on  block_type=assert
  buscreate : Subsystem  AncestorBlock=casper_library_flow_control/bus_create  mask(bus_create){inputNum=4}
      mask prompts: inputNum "Number of inputs:"
      mask init:
      | bus_create_init(gcb,...
      |     'inputNum', inputNum);
  io_delay : Subsystem  AncestorBlock=casper_library_delays/pipeline  mask(pipeline){csp_latency=2}
      mask prompts: csp_latency "Latency"
      mask help:
      | An explicitly laid-out delay line to avoid mapping to SRL16s
      | for use in pipelining to help achieve timing closure.
      mask init:
      | pipeline_init(gcb,'latency',csp_latency);
      settings: AttributesFormatString=Latency = %<latency>
      mask Display:
      | port_label('input', 1, 'd');
      | port_label('output', 1, 'q');
      | disp(['Z^-', num2str(csp_latency)]);
  ss : Subsystem  Tag=casper:snapshot  AncestorBlock=casper_library_scopes/snapshot  mask(snapshot){storage=bram, dram_dimm=2, dram_clock=250, nsamples=12, data_width=64, offset=off, circap=off, value=off, ext_arm=off, ext_circ=off, provide_outputs=off, use_dsp48=on}
      mask prompts: storage "Storage medium"; dram_dimm "DRAM dimm"; dram_clock "DRAM clock rate"; nsamples "Number of Samples (2^?)"; data_width "Data width"; offset "Start delay support"; circap "Circular capture support"; value "Extra value capture support"; ext_arm "External arm support"; ext_circ "External circular capture support"; provide_outputs "Provide outputs"; use_dsp48 "Use DSP48s to implement counters"
      mask help:
      | Standard snap block, but with the following optional extras;
      |  1) Optionally delay the fabric trigger by a user-specified number of valids.
      |  2) Capture continuously after a trigger until a stop pulse is received. Data is captured into BRAM continuously, with old data being overwritten until a stop command is received. Then stop capturing when memory is filled. This enables you to get some data before and some data after the stop pulse. Use the 'tr_en_cnt' register to determine where you are in your vector. 'Addr' register's MSb now indicates 'busy capturing'.
      |  3) Optionally capture a value on an input port to a register at the same time as the first data sample.
      |  4) Implement counters using DSP48Es to save resources.
      mask init:
      | snapshot_init(gcb, ...
      |     'storage', storage, ...
      |     'dram_dimm', dram_dimm, ...
      |     'dram_clock', dram_clock, ...
      |     'nsamples', nsamples, ...
      |     'data_width', data_width, ...
      |     'offset', offset, ...
      |     'circap', circap, ...
      |     'value', value, ...
      |     'ext_arm', ext_arm, ...
      |     'ext_circ', ext_circ, ...
      |     'provide_outputs', 'off', ...
      |     'use_dsp48', use_dsp48);
      settings: AttributesFormatString=|
      | 64 wide, 4096 deep
      | debugID: 125644504
      mask TypeOptions storage: bram | dram
      mask Callback storage: snapshot_callback();
      mask TypeOptions dram_dimm: 1 | 2 | 3 | 4
      mask TypeOptions dram_clock: 200 | 250 | 266 | 300 | 333
      mask TypeOptions data_width: 8 | 16 | 32 | 64 | 128
  trig_delay : Subsystem  AncestorBlock=casper_library_delays/pipeline  mask(pipeline){csp_latency=2}
      mask prompts: csp_latency "Latency"
      mask help:
      | An explicitly laid-out delay line to avoid mapping to SRL16s
      | for use in pipelining to help achieve timing closure.
      mask init:
      | pipeline_init(gcb,'latency',csp_latency);
      settings: AttributesFormatString=Latency = %<latency>
      mask Display:
      | port_label('input', 1, 'd');
      | port_label('output', 1, 'q');
      | disp(['Z^-', num2str(csp_latency)]);
  we_delay : Subsystem  AncestorBlock=casper_library_delays/pipeline  mask(pipeline){csp_latency=2}
      mask prompts: csp_latency "Latency"
      mask help:
      | An explicitly laid-out delay line to avoid mapping to SRL16s
      | for use in pipelining to help achieve timing closure.
      mask init:
      | pipeline_init(gcb,'latency',csp_latency);
      settings: AttributesFormatString=Latency = %<latency>
      mask Display:
      | port_label('input', 1, 'd');
      | port_label('output', 1, 'q');
      | disp(['Z^-', num2str(csp_latency)]);
  arm_out : Outport  VectorParamsAs1DForOutWhenUnconnected=off
  wires:
  ss/1(arm_out) -> arm_out/1
  buscreate/1(bus_out) -> io_delay/1(d)
  io_delay/1(q) -> ss/1(din)
  in_m00/1 -> assert_m00/1
  assert_m00/1 -> buscreate/1(in1)
  in_m10/1 -> assert_m10/1
  assert_m10/1 -> buscreate/2(in2)
  in_m20/1 -> assert_m20/1
  assert_m20/1 -> buscreate/3(in3)
  in_m30/1 -> assert_m30/1
  assert_m30/1 -> buscreate/4(in4)
  we/1 -> we_delay/1(d)
  we_delay/1(q) -> ss/2(we)
  trig/1 -> trig_delay/1(d)
  trig_delay/1(q) -> ss/3(trig)

== system test_rfdcmask_zcu216/counter_ctrl ==
  sim_1 : Inport
  convert1_1 : DataTypeConversion  OutDataTypeStr=fixdt('ufix32_En0')  LockScale=on
  convert2_1 : DataTypeConversion  OutDataTypeStr=fixdt('ufix32_En0')  ConvertRealWorld=Stored Integer (SI)  LockScale=on
  gain_1 : Gain
  io_delay : xbsIndex_r4/Delay  rst=off  infoeditControl=Selection of Reset will increase slice count due to use of real FFs and instead of SRLs  en=off  latency=0  reg_retiming=on  dbl_ovrd=off  block_type=delay
  reint1 : xbsIndex_r4/Reinterpret  force_arith_type=on  arith_type=Unsigned  force_bin_pt=on  bin_pt=0  block_type=reinterpret
  slice_reg : xbsIndex_r4/Slice  nbits=32  boolean_output=off  mode=Lower Bit Location + Width  bit1=0  base1=MSB of Input  bit0=0  base0=LSB of Input  dbl_ovrd=off  block_type=slice
  test_rfdcmask_zcu216_counter_ctrl_user_data_out : xbsIndex_r4/Gateway In  gui_display_data_type=Fixed-point  arith_type=Unsigned  n_bits=32  bin_pt=0  preci_type=Single  exp_width=8  frac_width=24  rows=1  columns=1  quantization="Round  (unbiased: +/- Inf)"  overflow=Saturate  period=1  UseAsADC=off  ADCChannel='1'  interface=None  automatic_assignment=on  address_offset=hex2dec('00')  intf_name=''  intf_description=''  default_value=0  timing_constraint=None  locs_specified=off  LOCs={}  io_standard={}  inherit_from_input=off  hdl_port=on  dbl_ovrd=off  block_type=gatewayin
  in_reg : Outport  VectorParamsAs1DForOutWhenUnconnected=off
  wires:
  test_rfdcmask_zcu216_counter_ctrl_user_data_out/1 -> io_delay/1
  sim_1/1 -> convert1_1/1
  convert1_1/1 -> convert2_1/1
  convert2_1/1 -> gain_1/1
  gain_1/1 -> test_rfdcmask_zcu216_counter_ctrl_user_data_out/1
  io_delay/1 -> slice_reg/1
  slice_reg/1 -> reint1/1
  reint1/1 -> in_reg/1

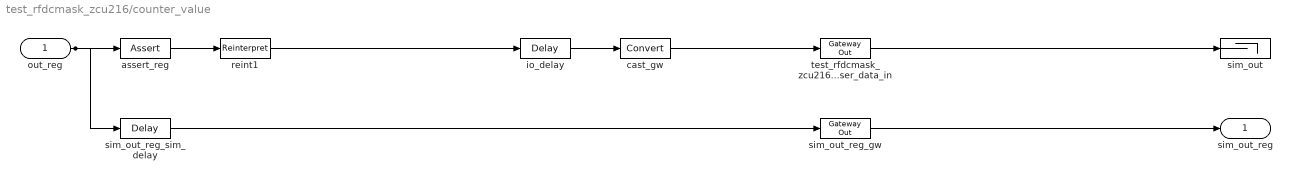
== system test_rfdcmask_zcu216/counter_value ==
  out_reg : Inport
  assert_reg : xbsIndex_r4/Assert  assert_type=on  type_source=Explicitly  gui_display_data_type=Fixed-point  arith_type=Unsigned  n_bits=32  bin_pt=0  preci_type=Single  exp_width=8  frac_width=24  assert_rate=off  rate_source=Explicitly  period=1  output_port=on  block_type=assert
  cast_gw : xbsIndex_r4/Convert  gui_display_data_type=Fixed-point  arith_type=Unsigned  n_bits=32  bin_pt=0  float_type=Single  exp_bits=8  fraction_bits=24  quantization=Truncate  overflow=Wrap  en=off  latency=1  pipeline=off  dbl_ovrd=off  block_type=convert
  io_delay : xbsIndex_r4/Delay  rst=off  infoeditControl=Selection of Reset will increase slice count due to use of real FFs and instead of SRLs  en=off  latency=0  reg_retiming=on  dbl_ovrd=off  block_type=delay
  reint1 : xbsIndex_r4/Reinterpret  force_arith_type=on  arith_type=Unsigned  force_bin_pt=on  bin_pt=0  block_type=reinterpret
  sim_out : Terminator
  sim_out_reg_gw : xbsIndex_r4/Gateway Out  inherit_from_input=off  hdl_port=off  rows=1  columns=1  UseAsDAC=off  DACChannel='1'  interface=None  automatic_assignment=on  address_offset=hex2dec('00')  intf_name=''  intf_description=''  timing_constraint=None  locs_specified=off  LOCs={}  io_standard={}  block_type=gatewayout
  sim_out_reg_sim_delay : xbsIndex_r4/Delay  rst=off  infoeditControl=Selection of Reset will increase slice count due to use of real FFs and instead of SRLs  en=off  latency=1  reg_retiming=on  dbl_ovrd=off  block_type=delay
  test_rfdcmask_zcu216_counter_value_user_data_in : xbsIndex_r4/Gateway Out  inherit_from_input=off  hdl_port=on  rows=1  columns=1  UseAsDAC=off  DACChannel='1'  interface=None  automatic_assignment=on  address_offset=hex2dec('00')  intf_name=''  intf_description=''  timing_constraint=None  locs_specified=off  LOCs={}  io_standard={}  block_type=gatewayout
  sim_out_reg : Outport  VectorParamsAs1DForOutWhenUnconnected=off
  wires:
  sim_out_reg_sim_delay/1 -> sim_out_reg_gw/1
  sim_out_reg_gw/1 -> sim_out_reg/1
  io_delay/1 -> cast_gw/1
  cast_gw/1 -> test_rfdcmask_zcu216_counter_value_user_data_in/1
  test_rfdcmask_zcu216_counter_value_user_data_in/1 -> sim_out/1
  out_reg/1 -> sim_out_reg_sim_delay/1, assert_reg/1
  assert_reg/1 -> reint1/1
  reint1/1 -> io_delay/1

== system test_rfdcmask_zcu216/gpio ==
  gpio_out : Inport
  convert : xbsIndex_r4/Convert  gui_display_data_type=Fixed-point  arith_type=Boolean  n_bits=1  bin_pt=0  float_type=Single  exp_bits=8  fraction_bits=24  quantization=Truncate  overflow=Wrap  en=off  latency=1  pipeline=off  dbl_ovrd=off  block_type=convert
  test_rfdcmask_zcu216_gpio_gateway : xbsIndex_r4/Gateway Out  inherit_from_input=off  hdl_port=on  rows=1  columns=1  UseAsDAC=off  DACChannel='1'  interface=None  automatic_assignment=on  address_offset=hex2dec('00')  intf_name=''  intf_description=''  timing_constraint=None  locs_specified=off  LOCs={}  io_standard={}  block_type=gatewayout
  sim_out : Outport  VectorParamsAs1DForOutWhenUnconnected=off
  wires:
  gpio_out/1 -> convert/1
  convert/1 -> test_rfdcmask_zcu216_gpio_gateway/1
  test_rfdcmask_zcu216_gpio_gateway/1 -> sim_out/1

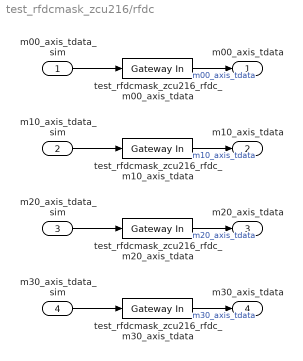
== system test_rfdcmask_zcu216/rfdc ==
  m00_axis_tdata_sim : Inport
  m10_axis_tdata_sim : Inport  Port=2
  m20_axis_tdata_sim : Inport  Port=3
  m30_axis_tdata_sim : Inport  Port=4
  test_rfdcmask_zcu216_rfdc_m00_axis_tdata : xbsIndex_r4/Gateway In  gui_display_data_type=Fixed-point  arith_type="Signed  (2's comp)"  n_bits=16  bin_pt=0  preci_type=Single  exp_width=8  frac_width=24  rows=1  columns=1  quantization="Round  (unbiased: +/- Inf)"  overflow=Saturate  period=1  UseAsADC=off  ADCChannel='1'  interface=None  automatic_assignment=on  address_offset=hex2dec('00')  intf_name=''  intf_description=''  default_value=0  timing_constraint=None  locs_specified=off  LOCs={}  io_standard={}  inherit_from_input=off  hdl_port=on  dbl_ovrd=off  block_type=gatewayin
  test_rfdcmask_zcu216_rfdc_m10_axis_tdata : xbsIndex_r4/Gateway In  gui_display_data_type=Fixed-point  arith_type="Signed  (2's comp)"  n_bits=16  bin_pt=0  preci_type=Single  exp_width=8  frac_width=24  rows=1  columns=1  quantization="Round  (unbiased: +/- Inf)"  overflow=Saturate  period=1  UseAsADC=off  ADCChannel='1'  interface=None  automatic_assignment=on  address_offset=hex2dec('00')  intf_name=''  intf_description=''  default_value=0  timing_constraint=None  locs_specified=off  LOCs={}  io_standard={}  inherit_from_input=off  hdl_port=on  dbl_ovrd=off  block_type=gatewayin
  test_rfdcmask_zcu216_rfdc_m20_axis_tdata : xbsIndex_r4/Gateway In  gui_display_data_type=Fixed-point  arith_type="Signed  (2's comp)"  n_bits=16  bin_pt=0  preci_type=Single  exp_width=8  frac_width=24  rows=1  columns=1  quantization="Round  (unbiased: +/- Inf)"  overflow=Saturate  period=1  UseAsADC=off  ADCChannel='1'  interface=None  automatic_assignment=on  address_offset=hex2dec('00')  intf_name=''  intf_description=''  default_value=0  timing_constraint=None  locs_specified=off  LOCs={}  io_standard={}  inherit_from_input=off  hdl_port=on  dbl_ovrd=off  block_type=gatewayin
  test_rfdcmask_zcu216_rfdc_m30_axis_tdata : xbsIndex_r4/Gateway In  gui_display_data_type=Fixed-point  arith_type="Signed  (2's comp)"  n_bits=16  bin_pt=0  preci_type=Single  exp_width=8  frac_width=24  rows=1  columns=1  quantization="Round  (unbiased: +/- Inf)"  overflow=Saturate  period=1  UseAsADC=off  ADCChannel='1'  interface=None  automatic_assignment=on  address_offset=hex2dec('00')  intf_name=''  intf_description=''  default_value=0  timing_constraint=None  locs_specified=off  LOCs={}  io_standard={}  inherit_from_input=off  hdl_port=on  dbl_ovrd=off  block_type=gatewayin
  m00_axis_tdata : Outport  VectorParamsAs1DForOutWhenUnconnected=off
  m10_axis_tdata : Outport  Port=2  VectorParamsAs1DForOutWhenUnconnected=off
  m20_axis_tdata : Outport  Port=3  VectorParamsAs1DForOutWhenUnconnected=off
  m30_axis_tdata : Outport  Port=4  VectorParamsAs1DForOutWhenUnconnected=off
  wires:
  m00_axis_tdata_sim/1 -> test_rfdcmask_zcu216_rfdc_m00_axis_tdata/1
  test_rfdcmask_zcu216_rfdc_m00_axis_tdata/1 -> m00_axis_tdata/1  "m00_axis_tdata"
  m10_axis_tdata_sim/1 -> test_rfdcmask_zcu216_rfdc_m10_axis_tdata/1
  test_rfdcmask_zcu216_rfdc_m10_axis_tdata/1 -> m10_axis_tdata/1  "m10_axis_tdata"
  m20_axis_tdata_sim/1 -> test_rfdcmask_zcu216_rfdc_m20_axis_tdata/1
  test_rfdcmask_zcu216_rfdc_m20_axis_tdata/1 -> m20_axis_tdata/1  "m20_axis_tdata"
  m30_axis_tdata_sim/1 -> test_rfdcmask_zcu216_rfdc_m30_axis_tdata/1
  test_rfdcmask_zcu216_rfdc_m30_axis_tdata/1 -> m30_axis_tdata/1  "m30_axis_tdata"

== system test_rfdcmask_zcu216/snapshot_ctrl ==
  sim_1 : Inport
  convert1_1 : DataTypeConversion  OutDataTypeStr=fixdt('ufix1_En0')  LockScale=on
  convert2_1 : DataTypeConversion  OutDataTypeStr=fixdt('ufix1_En0')  ConvertRealWorld=Stored Integer (SI)  LockScale=on
  gain_1 : Gain
  io_delay : xbsIndex_r4/Delay  rst=off  infoeditControl=Selection of Reset will increase slice count due to use of real FFs and instead of SRLs  en=off  latency=0  reg_retiming=on  dbl_ovrd=off  block_type=delay
  slice_start : xbsIndex_r4/Slice  nbits=1  boolean_output=on  mode=Lower Bit Location + Width  bit1=0  base1=MSB of Input  bit0=0  base0=LSB of Input  dbl_ovrd=off  block_type=slice
  test_rfdcmask_zcu216_snapshot_ctrl_user_data_out : xbsIndex_r4/Gateway In  gui_display_data_type=Fixed-point  arith_type=Unsigned  n_bits=32  bin_pt=0  preci_type=Single  exp_width=8  frac_width=24  rows=1  columns=1  quantization="Round  (unbiased: +/- Inf)"  overflow=Saturate  period=1  UseAsADC=off  ADCChannel='1'  interface=None  automatic_assignment=on  address_offset=hex2dec('00')  intf_name=''  intf_description=''  default_value=0  timing_constraint=None  locs_specified=off  LOCs={}  io_standard={}  inherit_from_input=off  hdl_port=on  dbl_ovrd=off  block_type=gatewayin
  in_start : Outport  VectorParamsAs1DForOutWhenUnconnected=off
  wires:
  test_rfdcmask_zcu216_snapshot_ctrl_user_data_out/1 -> io_delay/1
  sim_1/1 -> convert1_1/1
  convert1_1/1 -> convert2_1/1
  convert2_1/1 -> gain_1/1
  gain_1/1 -> test_rfdcmask_zcu216_snapshot_ctrl_user_data_out/1
  io_delay/1 -> slice_start/1
  slice_start/1 -> in_start/1
